simulink model "actuator"  (R2020b)
settings: Solver=VariableStepAuto  StartTime=0.0  StopTime=20  FixedStep=0.01  MaxStep=0.1  RelTol=1e-3  AbsTol=1e-3  SampleTimeConstraint=STIndependent  EnableMultiTasking=on
PreLoadFcn:
  | % Pressure source
  | p_source = 8e5; % Pa
  | 
  | % 4-way directional valve
  | valve_area_max = 3e-5; % m^2
  | L0 = 1e-5;
  | 
  | % Pipes
  | L_pipe = 20; % m
  | flow_area = 1e-4; % m^2
  | 
  | % Air muscle actuators
  | L_muscle = 30; % cm
  | L_braid = 32; % cm
  | n = 2.5;
  | 
  | % Flow control valves
  | dp_crack = 1e4; % Pa
  | dp_max = 2e4; % Pa
  | area_max = 1e-5; % m^2
  | area_leak = 1e-10; % m^2
  | area_restrict = 1e-6; % m^2
  | 
  | % Translational dampers
  | D_translation = 1; % N/(m/s)
  | 
  | % Translational hard stops
  | x_bound = 8; % cm
  | 
  | % Linkage
  | L_top = 15; % cm
  | L_bottom = 15; % cm
  | 
  | % Load
  | inertia = 0.005; % kg*m^2
  | D_rotation = 10; % N*m/(rad/s)
  | K_spring = 6.4; % N*m/rad
  | theta_upper = 0.4; % rad
  | theta_lower = 0; % rad
  | 
  | % Environment
  | T_atm = 293.15; % K
  | p_atm = 0.101325; % MPa
values from neighbouring files (symbols this model uses):
  anti_network = 0    [Para_in.m]
  network = 0    [Para_in.m]
libraries: fl_lib x22, SimscapeFluids_lib x8, fl_ps_legacy_lib x8, nesl_utility x5
(part 1 of 3)
CloseFcn:
  | try,close(h1_sscfluids_antagonistic_mckibben_actuator),end
  | clear h1_sscfluids_antagonistic_mckibben_actuator
  | try,close(h2_sscfluids_antagonistic_mckibben_actuator),end
  | clear h2_sscfluids_antagonistic_mckibben_actuator
  | 
  | clear simlog_sscfluids_antagonistic_mckibben_actuator tout
  | clear T_atm p_atm p_source flow_area
  | clear valve_area_max L0 L_pipe dp_crack dp_max
  | clear area_max area_leak area_restrict
  | clear L_muscle L_braid n D_translation x_bound
  | clear L_top L_bottom inertia D_rotation K_spring
  | clear theta_upper theta_lower
Description:
  | Antagonistic McKibben Muscle Actuator
settings Model: Tag=PublishSubsystemCustomStyle  Creator=The MathWorks, Inc.  LastModifiedBy=zhb
settings SolverCC: AutoScaleAbsTol=off
settings DataIOCC: MaxDataPoints=10000  ReturnWorkspaceOutputs=off  SignalLoggingName=logsout_sscfluids_antagonistic_mckibben_actuator
settings OptimizationCC: LifeSpan=inf
settings DebuggingCC: AllowSymbolicDim=off  PregeneratedLibrarySubsystemCodeDiagnostic=none  SFUnexpectedBacktrackingDiag=warning  SFNoUnconditionalDefaultTransitionDiag=warning  SFExecutionAtInitializationDiag=none  ArithmeticOperatorsInVariantConditions=warning
settings SFSimCC: SimUseLocalCustomCode=off  CustomCodeUndefinedFunction=UseInterfaceOnly
settings RTWCC: RTWUseLocalCustomCode=off
settings CodeAppCC: StateflowObjectComments=on
settings GRTTargetCC: TargetLangStandard=C89/C90 (ANSI)
settings ConfigComp: CovMetricSettings=dw  CovSaveCumulativeToWorkspaceVar=on  CovSaveSingleToWorkspaceVar=on  CovExternalEMLEnable=off  CovSFcnEnable=off
settings SimscapeCC: SimscapeLogType=all  SimscapeLogSimulationStatistics=on  SimscapeLogName=simlog_sscfluids_antagonistic_mckibben_actuator  SimscapeLogLimitData=off  SimscapeLogDataHistory=10000

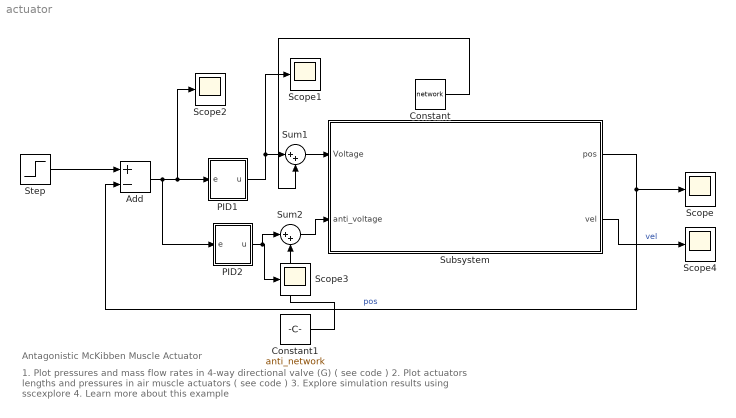
== system actuator ==
  note: Antagonistic McKibben Muscle Actuator
  note: 1. Plot pressures and mass flow rates in 4-way directional valve (G) ( see code )
      | 2. Plot actuators lengths and pressures in air muscle actuators ( see code )
      | 3. Explore simulation results using sscexplore
      | 4. Learn more about this example
  Add : Sum  Inputs=+-
  Constant : Constant  Value=network
  Constant1 : Constant  Value=anti_network
  PID1 : Subsystem  mask{Kc=-0.800, Td=0.0, Ti=14.700, Ad=10, U0=0}
      mask Display: disp('PID(s)')
  PID2 : Subsystem  mask{Kc=0.600, Td=0.0, Ti=14.700, Ad=10, U0=0}
      mask Display: disp('PID(s)')
  Scope{,1..4} (5 alike) : Scope
  Step : Step  Time=5  After=10  SampleTime=0
  Subsystem : Subsystem
  Sum1 : Sum  Inputs=|++
  Sum2 : Sum  Inputs=|++
  wires:
  PID1/1("u ") -> Sum1/1, Scope1/1
  Add/1 -> PID2/1(e), Scope2/1, PID1/1(e)
  Step/1 -> Add/1
  Subsystem/1(pos) -> Add/2, Scope/1  "pos"
  PID2/1("u ") -> Sum2/1, Scope3/1
  Subsystem/2(vel) -> Scope4/1  "vel"
  Sum1/1 -> Subsystem/1(Voltage)
  Constant/1 -> Sum1/2
  Sum2/1 -> Subsystem/2(anti_voltage)
  Constant1/1 -> Sum2/2

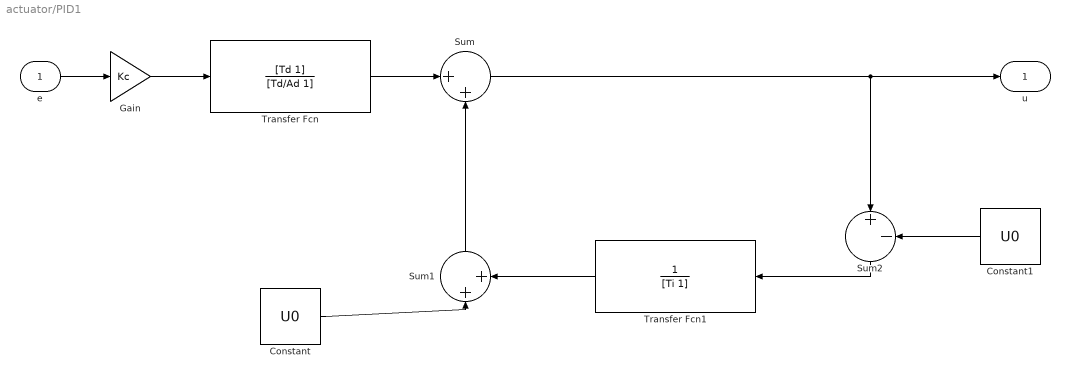
== system actuator/PID1 ==
  e : Inport
  Constant : Constant  Value=U0
  Constant1 : Constant  Value=U0
  Gain : Gain  Gain=Kc
  Sum : Sum  Inputs=|++
  Sum1 : Sum  Inputs=|++
  Sum2 : Sum  Inputs=|+-
  Transfer Fcn : TransferFcn  Numerator=[Td 1]  Denominator=[Td/Ad 1]
  Transfer Fcn1 : TransferFcn  Denominator=[Ti 1]
  "u " : Outport  VectorParamsAs1DForOutWhenUnconnected=off
  wires:
  e/1 -> Gain/1
  Constant/1 -> Sum1/1
  Gain/1 -> Transfer Fcn/1
  Transfer Fcn1/1 -> Sum1/2
  Transfer Fcn/1 -> Sum/1
  Sum1/1 -> Sum/2
  Sum/1 -> "u "/1, Sum2/1
  Constant1/1 -> Sum2/2
  Sum2/1 -> Transfer Fcn1/1

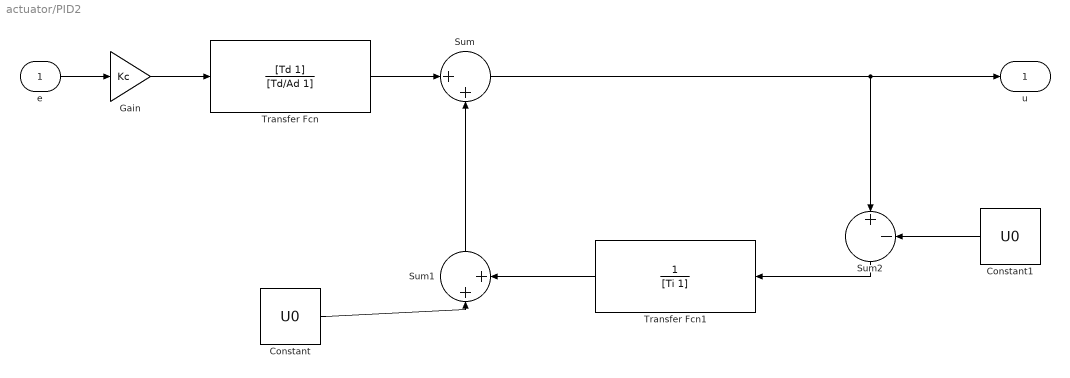
== system actuator/PID2 ==
  e : Inport
  Constant : Constant  Value=U0
  Constant1 : Constant  Value=U0
  Gain : Gain  Gain=Kc
  Sum : Sum  Inputs=|++
  Sum1 : Sum  Inputs=|++
  Sum2 : Sum  Inputs=|+-
  Transfer Fcn : TransferFcn  Numerator=[Td 1]  Denominator=[Td/Ad 1]
  Transfer Fcn1 : TransferFcn  Denominator=[Ti 1]
  "u " : Outport  VectorParamsAs1DForOutWhenUnconnected=off
  wires:
  e/1 -> Gain/1
  Constant/1 -> Sum1/1
  Gain/1 -> Transfer Fcn/1
  Transfer Fcn1/1 -> Sum1/2
  Transfer Fcn/1 -> Sum/1
  Sum1/1 -> Sum/2
  Sum/1 -> "u "/1, Sum2/1
  Constant1/1 -> Sum2/2
  Sum2/1 -> Transfer Fcn1/1
